simulink subsystem "Send_Actuator_Cmds_eSPAARO5"  (R2025a)
settings: Solver=VariableStepAuto  StartTime=0.0  StopTime=10.0  RelTol=1e-3
libraries: px4Peripheralslib x2
settings Model: Creator=gurt1  LastModifiedBy=gurt1
settings RTWCC: GPUComputeCapability=3.5

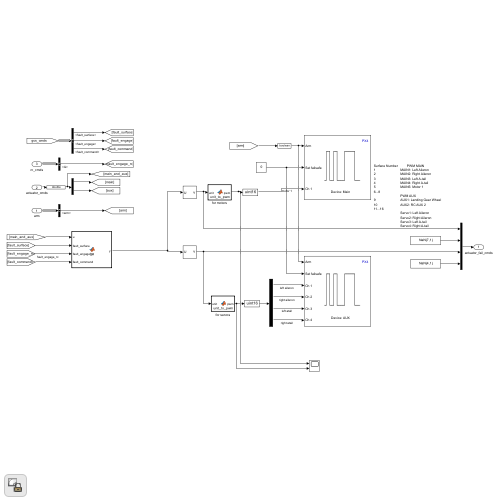
[thumbnail: Simulink's stored preview of the top-level diagram]
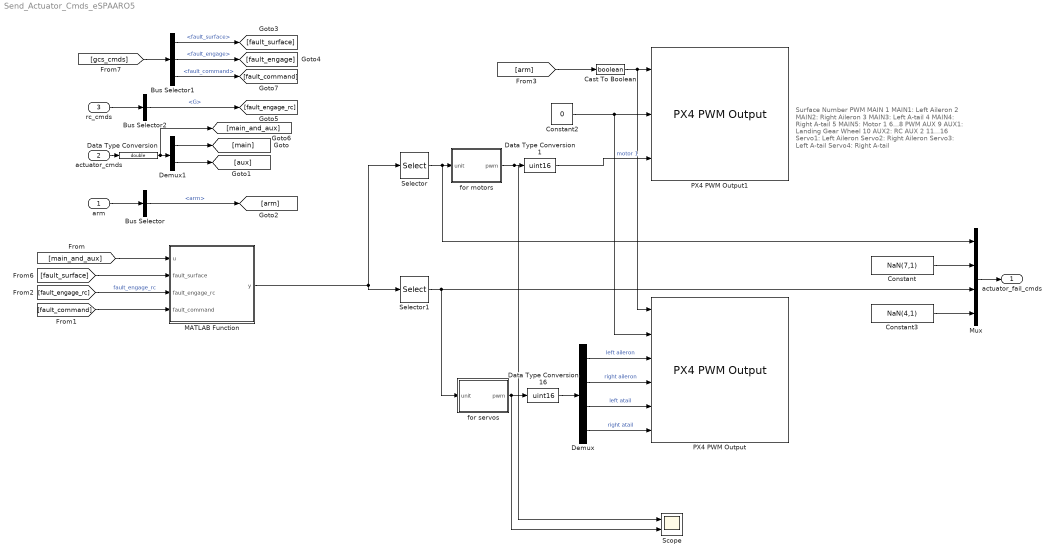
== system Send_Actuator_Cmds_eSPAARO5 ==
  note: Surface Number   	PWM MAIN
      | 1				MAIN1: Left Aileron
      | 2				MAIN2: Right Aileron
      | 3				MAIN3: Left A-tail
      | 4				MAIN4: Right A-tail
      | 5				MAIN5: Motor 1
      | 6...8
      | 				PWM AUX
      | 9				AUX1: Landing Gear Wheel
      | 10				AUX2: RC AUX 2
      | 11...16
      | 				Servo1: Left Aileron
      | 				Servo2: Right Aileron
      | 				Servo3: Left A-tail
      | 				Servo4: Right A-tail
  arm : Inport
  actuator_cmds : Inport  Port=2
  rc_cmds : Inport  Port=3
  Bus Selector : BusSelector  OutputSignals=arm
  Bus Selector1 : BusSelector  OutputSignals=Fault.fault_surface,Fault.fault_engage,Fault.fault_command
  Bus Selector2 : BusSelector  OutputSignals=switches.G
  Cast To Boolean : DataTypeConversion  OutDataTypeStr=boolean  SaturateOnIntegerOverflow=off  RndMeth=Floor
  Constant : Constant  Value=NaN(7,1)  OutDataTypeStr=double  SampleTime=-1
  Constant2 : Constant  Value=0  OutDataTypeStr=boolean  SampleTime=-1
  Constant3 : Constant  Value=NaN(4,1)  OutDataTypeStr=double  SampleTime=-1
  Data Type Conversion : DataTypeConversion  OutDataTypeStr=double  SaturateOnIntegerOverflow=off  RndMeth=Floor
  Data Type Conversion1 : DataTypeConversion  OutDataTypeStr=uint16  SaturateOnIntegerOverflow=off  RndMeth=Floor
  Data Type Conversion16 : DataTypeConversion  OutDataTypeStr=uint16  SaturateOnIntegerOverflow=off  RndMeth=Floor
  Demux : Demux
  Demux1 : Demux  Outputs=[8 8]
  MATLAB Function : MATLAB Function  TreatAsAtomicUnit=on
  Mux : Mux
  PX4 PWM Output : px4Peripheralslib/PX4 PWM Output  pwmDevice=AUX  pwmChannel1_=on  pwmChannel2_=on  pwmChannel3_=on  pwmChannel4_=on  pwmChannel5_=off  pwmChannel6_=off  pwmChannel7_=off  pwmChannel8_=off
  PX4 PWM Output1 : px4Peripheralslib/PX4 PWM Output  pwmDevice=Main  pwmChannel1_=on  pwmChannel2_=off  pwmChannel3_=off  pwmChannel4_=off  pwmChannel5_=off  pwmChannel6_=off  pwmChannel7_=off  pwmChannel8_=off
  Scope : Scope  NumInputPorts=2
      settings: ActiveDisplayYMinimum=356.82364721167937  ActiveDisplayYMaximum=1788.5871750948861  DataLoggingVariableName=ScopeData2
  Selector : Selector  InputPortWidth=16  IndexOptions=Index vector (dialog)  Indices=[1]  OutputSizes=1
  Selector1 : Selector  InputPortWidth=16  IndexOptions=Index vector (dialog)  Indices=[9:12]  OutputSizes=1
  for motors : MATLAB Function  TreatAsAtomicUnit=on
  for servos : MATLAB Function  TreatAsAtomicUnit=on
  actuator_fail_cmds : Outport
  wires:
  Constant3/1 -> Mux/4
  Constant/1 -> Mux/2
  Selector1/1 -> for servos/1(unit), Mux/3
  Selector/1 -> for motors/1(unit), Mux/1
  actuator_cmds/1 -> Data Type Conversion/1
  [arm] -> Cast To Boolean/1
  [main_and_aux] -> MATLAB Function/1(u)
  for motors/1(pwm) -> Scope/1, Data Type Conversion1/1
  arm/1 -> Bus Selector/1
  Bus Selector/1 -> [arm]  "<arm>"
  [gcs_cmds] -> Bus Selector1/1
  Bus Selector1/1 -> [fault_surface]  "<fault_surface>"
  Bus Selector1/2 -> [fault_engage]  "<fault_engage>"
  [fault_surface] -> MATLAB Function/2(fault_surface)
  Mux/1 -> actuator_fail_cmds/1
  rc_cmds/1 -> Bus Selector2/1
  Bus Selector2/1 -> [fault_engage_rc]  "<G>"
  [fault_engage_rc] -> MATLAB Function/3(fault_engage_rc)  "fault_engage_rc"
  Cast To Boolean/1 -> PX4 PWM Output/1, PX4 PWM Output1/1
  Constant2/1 -> PX4 PWM Output1/2, PX4 PWM Output/2
  Data Type Conversion16/1 -> Demux/1
  for servos/1(pwm) -> Scope/2, Data Type Conversion16/1
  MATLAB Function/1(y) -> Selector/1, Selector1/1
  Demux1/1 -> [main]
  Data Type Conversion1/1 -> PX4 PWM Output1/3  "motor 1"
  Demux/4 -> PX4 PWM Output/6  "right atail"
  Demux/3 -> PX4 PWM Output/5  "left atail"
  Demux/2 -> PX4 PWM Output/4  "right aileron"
  Demux/1 -> PX4 PWM Output/3  "left aileron"
  Demux1/2 -> [aux]
  Data Type Conversion/1 -> Demux1/1, [main_and_aux]
  Bus Selector1/3 -> [fault_command]  "<fault_command>"
  [fault_command] -> MATLAB Function/4(fault_command)

== matlab function Send_Actuator_Cmds_eSPAARO5/MATLAB Function ==
  data: u input; fault_surface input; y output; fault_engage_rc input; fault_command input
function y = fcn(u, fault_surface, fault_engage_rc, fault_command)

if fault_engage_rc == 0% || fault_engage == 1
    u(fault_surface) = fault_command;
    y = u;
else
    y = u;
end

== matlab function Send_Actuator_Cmds_eSPAARO5/for servos ==
  data: unit input; pwm output
%% unit_to_pwm
% DESCRIPTION: 
%   This function reads in a vector and maps the input from 0 to 1 to the range 
%   of 1000 to 2000. It also checks if any input values are -1 or NaN, and if so, 
%   sets the corresponding output value to 800.
%
% INPUTS: 
%   u   - (Nx1) Input vector with values to be mapped
%
% OUTPUTS:
%   y   - (Nx1) Output vector with mapped PWM values (1000 to 2000 or 800 for invalid inputs)
% 
% WRITTEN BY:
%   Garrett D. Asper
%   Virginia Tech
%   Email: garrettasper@vt.edu
%
% HISTORY:
%   16 SEP 2024 - Created and debugged, GDA
%
% NOMENCLATURE:                                  UNITS:
%   Not Applicable                                  Not Applicable

function pwm = unit_to_pwm(unit)

    % Map the input from 0 to 1 to 1000 to 2000
    unit = (unit+1)./2;
    pwm = unit*1000 + 1000;

    % Iterate through each value to apply constraints
    for i = 1:length(pwm)
        if isnan(unit(i)) || unit(i) == -1
            % Set the output to 800 for invalid inputs (-1 or NaN)
            pwm(i) = 800;
        elseif pwm(i) > 2000
            pwm(i) = 2000;
        elseif pwm(i) < 1000
            pwm(i) = 1000;
        end
    end

end

== matlab function Send_Actuator_Cmds_eSPAARO5/for motors ==
  data: unit input; pwm output
%% unit_to_pwm
% DESCRIPTION: 
%   This function reads in a vector and maps the input from 0 to 1 to the range 
%   of 1000 to 2000. It also checks if any input values are -1 or NaN, and if so, 
%   sets the corresponding output value to 800.
%
% INPUTS: 
%   u   - (Nx1) Input vector with values to be mapped
%
% OUTPUTS:
%   y   - (Nx1) Output vector with mapped PWM values (1000 to 2000 or 800 for invalid inputs)
% 
% WRITTEN BY:
%   Garrett D. Asper
%   Virginia Tech
%   Email: garrettasper@vt.edu
%
% HISTORY:
%   16 SEP 2024 - Created and debugged, GDA
%
% NOMENCLATURE:                                  UNITS:
%   Not Applicable                                  Not Applicable

function pwm = unit_to_pwm(unit)

    % Map the input from 0 to 1 to 1000 to 2000
    pwm = unit*1000 + 1000;

    % Iterate through each value to apply constraints
    for i = 1:length(pwm)
        if isnan(unit(i)) || unit(i) == -1
            % Set the output to 800 for invalid inputs (-1 or NaN)
            pwm(i) = 500;
        elseif pwm(i) > 1900
            pwm(i) = 1900;
        elseif pwm(i) < 1100
            pwm(i) = 1100;
        end
    end

end
